simulink model "AdaptiveThresholdSigmaDelta"  (R2020a)
settings: Solver=VariableStepAuto  StartTime=0.0  StopTime=10  RelTol=1e-3
undefined symbols (not defined in the file): DiscIntNeverNeededParam
libraries: dspfdesign x1
settings Model: Creator=diflo  LastModifiedBy=diflo

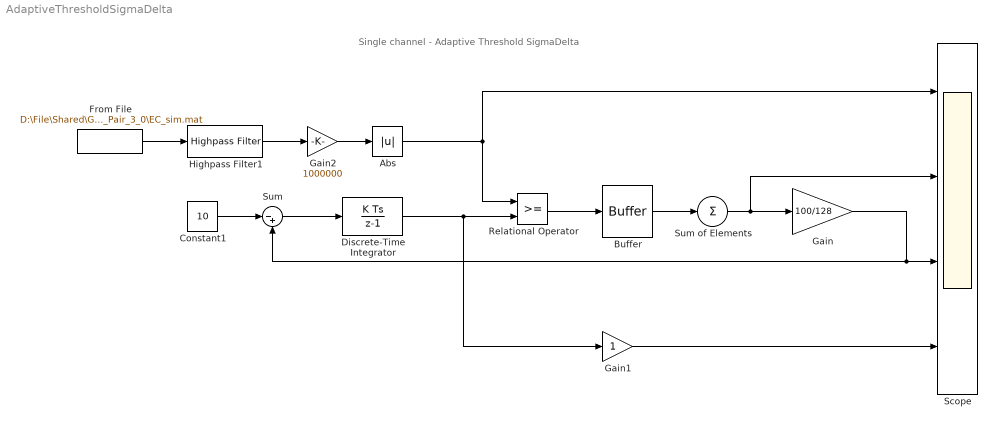
== system AdaptiveThresholdSigmaDelta ==
  note: Single channel - Adaptive Threshold SigmaDelta
  Abs : Abs
  Buffer : Buffer  N=128  OutputFrames=off
  Constant1 : Constant  Value=10  SampleTime=1/30000
  Discrete-Time Integrator : DiscreteIntegrator  gainval=0.1  SampleTime=1/30000  ICPrevOutput=DiscIntNeverNeededParam  ICPrevScaledInput=DiscIntNeverNeededParam
  From File : FromFile  FileName=D:\File\Shared\Google Drive\IIT - Neuroengineering\Project\WP1\Data\KampffLab\2014_11_25_Pair_3_0\EC_sim.mat  SampleTime=1/30000
  Gain : Gain  Gain=100/128
  Gain1 : Gain
  Gain2 : Gain  Gain=1000000
  Highpass Filter1 : dspfdesign/Highpass Filter  FilterType=IIR  DesignForMinimumOrder=off  FilterOrder=3  StopbandFrequency=1  PassbandFrequency=300  StopbandAttenuation=80  PassbandRipple=0.1  InheritSampleRate=off  SampleRate=30000  SimulateUsing=Interpreted execution  roundingMode=Floor  coeffsDataTypeStr=fixdt(1,16)
  Relational Operator : RelationalOperator  OutDataTypeStr=boolean
  Scope : Scope  NumInputPorts=4
  Sum : Sum  Inputs=|-+
  Sum of Elements : Sum  Inputs=+
  wires:
  Abs/1 -> Scope/1, Relational Operator/1
  Discrete-Time Integrator/1 -> Gain1/1, Relational Operator/2
  Sum/1 -> Discrete-Time Integrator/1
  Constant1/1 -> Sum/1
  Relational Operator/1 -> Buffer/1
  Buffer/1 -> Sum of Elements/1
  Sum of Elements/1 -> Scope/2, Gain/1
  Gain/1 -> Sum/2, Scope/3
  Gain1/1 -> Scope/4
  From File/1 -> Highpass Filter1/1
  Highpass Filter1/1 -> Gain2/1
  Gain2/1 -> Abs/1
